simulink model "Controle_SISO"  (R2021a)
settings: Solver=VariableStepAuto  StartTime=0.0  StopTime=200  RelTol=1e-3
libraries: pid_lib x1, simulink x1
settings Model: Creator=Aula  LastModifiedBy=Aula

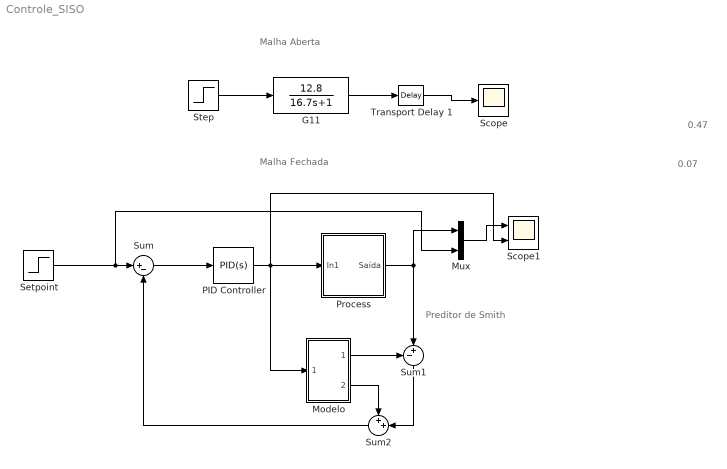
== system Controle_SISO ==
  note: Preditor de Smith
  note: 0.07
  note: 0.47
  note: Malha Aberta
  note: Malha Fechada
  G11 : TransferFcn  Numerator=[12.8]  Denominator=[16.7 1]
  Modelo : Subsystem
  Mux : Mux  Inputs=2
  "PID Controller " : pid_lib/PID Controller  Controller=PID  Form=Parallel  TimeDomain=Continuous-time  UseExternalTs=off  SampleTime=-1  IntegratorMethod=Forward Euler  FilterMethod=Forward Euler  ControllerParametersSource=internal  P=0.47  I=0.07  D=0  UseFilter=on  N=100  TunerSelectOption=Transfer Function Based (PID Tuner App)  InitialConditionSource=internal  InitialConditionForIntegrator=0  InitialConditionForFilter=0  DifferentiatorICPrevScaledInput=0  ExternalReset=none  TrackingMode=off  Kt=1  LimitOutput=off  SatLimitsSource=internal  UpperSaturationLimit=inf  LowerSaturationLimit=-inf  LinearizeAsGain=on  AntiWindupMode=none  Kb=1  POutMin=[]  POutMax=[]  IOutMin=[]  IOutMax=[]  DOutMin=[]  DOutMax=[]  NOutMin=[]  NOutMax=[]  SumOutMin=[]  SumOutMax=[]  SaturationOutMin=[]  SaturationOutMax=[]  PParamMin=[]  PParamMax=[]  IParamMin=[]  IParamMax=[]  DParamMin=[]  DParamMax=[]  NParamMin=[]  NParamMax=[]  KbParamMin=[]  KbParamMax=[]  KtParamMin=[]  KtParamMax=[]  KbOutMin=[]  KbOutMax=[]  KtOutMin=[]  KtOutMax=[]  IntegratorOutMin=[]  IntegratorOutMax=[]  FilterOutMin=[]  FilterOutMax=[]  SumI1OutMin=[]  SumI1OutMax=[]  SumI2OutMin=[]  SumI2OutMax=[]  SumI3OutMin=[]  SumI3OutMax=[]  SumI4OutMin=[]  SumI4OutMax=[]  SumDOutMin=[]  SumDOutMax=[]  DifferentiatorOutMin=[]  DifferentiatorOutMax=[]  FilterDiffOutCoefMin=[]  FilterDiffOutCoefMax=[]  ReciprocalOutMin=[]  ReciprocalOutMax=[]  SumDenOutMin=[]  SumDenOutMax=[]  SumNumOutMin=[]  SumNumOutMax=[]  DivideOutMin=[]  DivideOutMax=[]  UdiffTsProdOutMin=[]  UdiffTsProdOutMax=[]  NTsProdOutMin=[]  NTsProdOutMax=[]  UintegralTsProdOutMin=[]  UintegralTsProdOutMax=[]  UngainTsProdOutMin=[]  UngainTsProdOutMax=[]  IntegratorContinuousStateAttributes=''  IntegratorStateMustResolveToSignalObject=off  IntegratorRTWStateStorageClass=Auto  FilterContinuousStateAttributes=''  FilterStateMustResolveToSignalObject=off  FilterRTWStateStorageClass=Auto  ParallelPVariant=InternalParameters  IdealPVariant=Disabled  IVariant=InternalParameters  DVariant=InternalParameters  IntegratorVariant=Continuous  SatVariant=Disabled  AWVariant=Passthrough  PCopyVariant=Disabled  TRVariant=Disabled  FdbkBlocksVariant=Forward  IdealPFdbkVariant=Disabled  SatFdbkVariant=Disabled  DerivativeFilterVariant=ContFilter  NVariant=InternalParameters  NCopyVariant=Disabled  FilterICVariant=InternalICsFilter  IntegratorICVariant=InternalICs  ExternalResetVariant=Disabled  TRSumVariant=Passthrough  SumFdbkVariant=Disabled  SumVariant=Sum_PID  TsampFilterVariant=InternalTs  TsampNgainVariant=Passthrough  TsampIntegralVariant=Passthrough  ExternalSaturationOutDataTypeStr=Inherit: Same as second input
  Process : Subsystem
  Scope : Scope
  Scope1 : Scope  NumInputPorts=2
  Setpoint : Step  Time=10  SampleTime=0
  Step : Step  SampleTime=0
  Sum : Sum  Inputs=|+-
  Sum1 : Sum  Inputs=-+|
  Sum2 : Sum  Inputs=++|
  Transport Delay 1 : TransportDelay
  wires:
  Step/1 -> G11/1
  G11/1 -> Transport Delay 1/1
  "PID Controller "/1 -> Modelo/1(In1), Process/1(In1), Scope1/2
  Sum/1 -> "PID Controller "/1
  Setpoint/1 -> Mux/2, Sum/1
  Mux/1 -> Scope1/1
  Transport Delay 1/1 -> Scope/1
  Modelo/1(ym) -> Sum1/1
  Modelo/2(ymr) -> Sum2/1
  Sum1/1 -> Sum2/2
  Sum2/1 -> Sum/2
  Process/1(Saída) -> Mux/1, Sum1/2

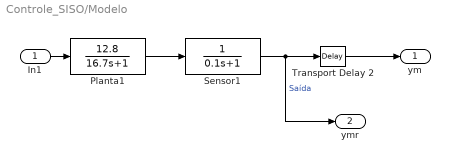
== system Controle_SISO/Modelo ==
  In1 : Inport
  Planta1 : TransferFcn  Numerator=[12.8]  Denominator=[16.7 1]
  Sensor1 : TransferFcn  Denominator=[0.1 1]
  Transport Delay 2 : TransportDelay  DelayTime=5
  ym : Outport
  ymr : Outport  Port=2
  wires:
  Planta1/1 -> Sensor1/1
  Sensor1/1 -> ymr/1, Transport Delay 2/1  "Saída"
  In1/1 -> Planta1/1
  Transport Delay 2/1 -> ym/1

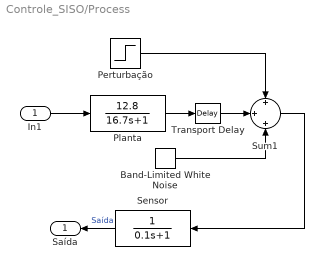
== system Controle_SISO/Process ==
  In1 : Inport
  Band-Limited White Noise : simulink/Sources/Band-Limited White Noise  Cov=[1e-4]  Ts=0.1  seed=[23341]
  Perturbação : Step  Time=100  After=0.5  SampleTime=0
  Planta : TransferFcn  Numerator=[12.8]  Denominator=[16.7 1]
  Sensor : TransferFcn  Denominator=[0.1 1]
  Sum1 : Sum  Inputs=+|+|+
  "Transport Delay " : TransportDelay  DelayTime=5
  Saída : Outport
  wires:
  In1/1 -> Planta/1
  Sensor/1 -> Saída/1  "Saída"
  Planta/1 -> "Transport Delay "/1
  Perturbação/1 -> Sum1/1
  "Transport Delay "/1 -> Sum1/2
  Band-Limited White Noise/1 -> Sum1/3
  Sum1/1 -> Sensor/1
